simulink model "chris_1R_hsv_vortex_follow"  (R2024b)
settings: Solver=FixedStepDiscrete  StartTime=0.0  StopTime=20  FixedStep=0.1  MaxStep=0.1  RelTol=1e-3
libraries: realtime_pacer_lib x1
settings Model: Creator=RSL  LastModifiedBy=cwaight
settings SolverCC: AlgebraicLoopSolver=TrustRegion
settings DataIOCC: ReturnWorkspaceOutputs=off
settings DebuggingCC: UnconnectedInputMsg=warning  UnconnectedOutputMsg=warning  UnconnectedLineMsg=warning  ArithmeticOperatorsInVariantConditions=warning
settings ModelReferenceCC: EnableRefExpFcnMdlSchedulingChecks=on
settings SFSimCC: SimUseLocalCustomCode=off  CustomCodeUndefinedFunction=UseInterfaceOnly
settings RTWCC: RTWUseLocalCustomCode=off  GPUComputeCapability=3.5
settings CodeAppCC: StateflowObjectComments=on

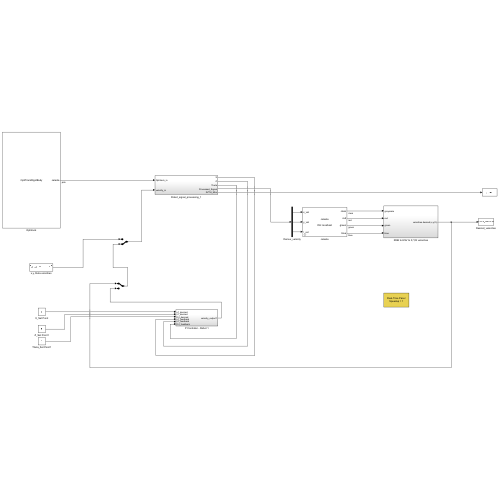
[thumbnail: Simulink's stored preview of the top-level diagram]
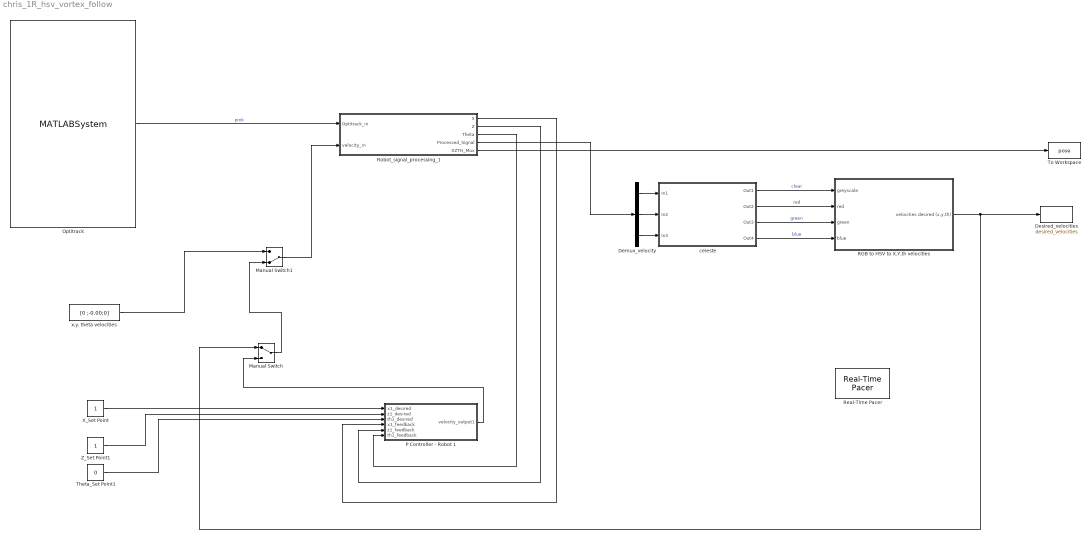
== system chris_1R_hsv_vortex_follow ==
  Demux_velocity : Demux  Outputs=3
  Desired_velocities : ToWorkspace  VariableName=desired_velocities  SampleTime=-1
  Manual Switch : ManualSwitch
  Manual Switch1 : ManualSwitch  CurrentSetting=0
  Optitrack : MATLABSystem  System=OptiTrackRigidBody  coordinateTransformationMatrix=[ 1, 0, 0; 0, 0, 1; 0, -1, 0 ]  rigidBodyNames={ 'celeste'}  orientationFormat=Euler angles  debug=on  natNetHostAddress=127.0.0.1  natNetClientAddress=127.0.0.1  dllPath=C:\DecaMATLAB\NatNetSDK\lib\x64\NatNetML.dll  unicast=off
      mask Type: OptiTrackRigidBody
      mask Display:
      | disp('OptiTrackRigidBody');
      | port_label('output',1,'celeste');
  P Controller - Robot 1 : Subsystem
  RGB to HSV to X,Y,th velocities : Subsystem
  Real-Time Pacer : realtime_pacer_lib/Real-Time Pacer  simTimePerRealTime=1
  Robot_signal_processing_1 : Subsystem
  "Theta_Set Point1 " : Constant  Value=0
  To Workspace : ToWorkspace  VariableName=pose  SampleTime=-1
  X_Set Point : Constant
  Z_Set Point1 : Constant
  celeste : Subsystem  mask(DecabotMask){robotName=celeste, decabotHelper=localhost, robotAddress=, useDataTurbine=off, useDirectSocket=on, debug=off}
      mask prompts: robotName "Robot name:"; decabotHelper "DecabotHelper/DataTurbine server:"; robotAddress "Robot network address (optional):"; useDataTurbine "Use DataTurbine"; useDirectSocket "Use direct robot TCP connection"; debug "Log debug messages"
      mask help: This is a masked subsystem that contains a Decabot block for bidirectional communication with a decabot over a direct TCP socket connection.
      mask init:
      | robotName = 'Nobody';
      | decabotHelper = 'localhost';
      | robotAddress = '';
      | useDataTurbine = true;
      | debug = true;
      mask TypeOptions robotName: decabot/robotName
      mask Callback robotName:
      | try
      |     set_param( gcb( ), 'Name', get_param( gcb( ), 'robotName' ) );
      | end
      mask TypeOptions decabotHelper: decabot/decabotHelper
      mask TypeOptions robotAddress: decabot/robotAddress
      mask TypeOptions useDataTurbine: decabot/useDataTurbine
      mask TypeOptions useDirectSocket: decabot/useDirectSocket
      mask TypeOptions debug: decabot/debug
      mask Display:
      | disp( [get_param( gcb( ), 'robotName' ) '\n\nDH: ' get_param( gcb( ), 'decabotHelper' ) ] );
      | 
      | port_label('input',1,'x_vel');
      | port_label('input',2,'y_vel');
      | port_label('input',3,'t_vel');
      | 
      | port_label('output',1,'clear');
      | port_label('output',2,'red');
      | port_label('output',3,'green');
      | port_label('output',4,'blue');
  "x,y, theta velocities" : Constant  Value=[0 ;-0.00;0]
  wires:
  Demux_velocity/3 -> celeste/3(In3)
  Demux_velocity/1 -> celeste/1(In1)
  Demux_velocity/2 -> celeste/2(In2)
  X_Set Point/1 -> P Controller - Robot 1/1(x1_desired)
  Z_Set Point1/1 -> P Controller - Robot 1/2(z1_desired)
  "Theta_Set Point1 "/1 -> P Controller - Robot 1/3(th1_desired)
  Robot_signal_processing_1/3(Theta) -> P Controller - Robot 1/6(th1_feedback)
  Robot_signal_processing_1/2(Z) -> P Controller - Robot 1/5(z1_feedback)
  Robot_signal_processing_1/1(X) -> P Controller - Robot 1/4(x1_feedback)
  Optitrack/1 -> Robot_signal_processing_1/1(Optitrack_in)  "pink"
  Robot_signal_processing_1/4(Processed_Signal) -> Demux_velocity/1
  celeste/1(Out1) -> RGB to HSV to X,Y,th velocities/1(greyscale)  "clear"
  celeste/2(Out2) -> RGB to HSV to X,Y,th velocities/2(red)  "red"
  celeste/3(Out3) -> RGB to HSV to X,Y,th velocities/3(green)  "green"
  celeste/4(Out4) -> RGB to HSV to X,Y,th velocities/4(blue)  "blue"
  Manual Switch1/1 -> Robot_signal_processing_1/2(velocity_in)
  P Controller - Robot 1/1(velocity_output1) -> Manual Switch/2
  Manual Switch/1 -> Manual Switch1/2
  "x,y, theta velocities"/1 -> Manual Switch1/1
  RGB to HSV to X,Y,th velocities/1(velocities desired (x,y,th)) -> Desired_velocities/1, Manual Switch/1
  Robot_signal_processing_1/5(XZTH_Mux) -> To Workspace/1

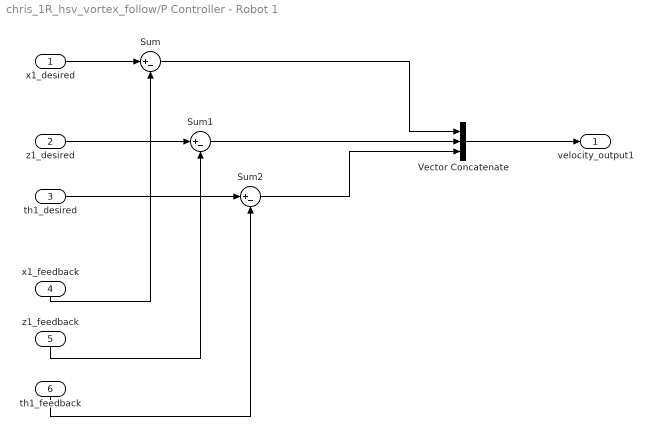
== system chris_1R_hsv_vortex_follow/P Controller - Robot 1 ==
  x1_desired : Inport
  z1_desired : Inport  Port=2
  th1_desired : Inport  Port=3
  x1_feedback : Inport  Port=4
  z1_feedback : Inport  Port=5
  th1_feedback : Inport  Port=6
  Sum : Sum  Inputs=|+-
  Sum1 : Sum  Inputs=|+-
  Sum2 : Sum  Inputs=|+-
  Vector Concatenate : Concatenate  NumInputs=3
  velocity_output1 : Outport
  wires:
  Vector Concatenate/1 -> velocity_output1/1
  x1_desired/1 -> Sum/1
  Sum/1 -> Vector Concatenate/1
  th1_feedback/1 -> Sum2/2
  x1_feedback/1 -> Sum/2
  z1_feedback/1 -> Sum1/2
  Sum2/1 -> Vector Concatenate/3
  th1_desired/1 -> Sum2/1
  Sum1/1 -> Vector Concatenate/2
  z1_desired/1 -> Sum1/1

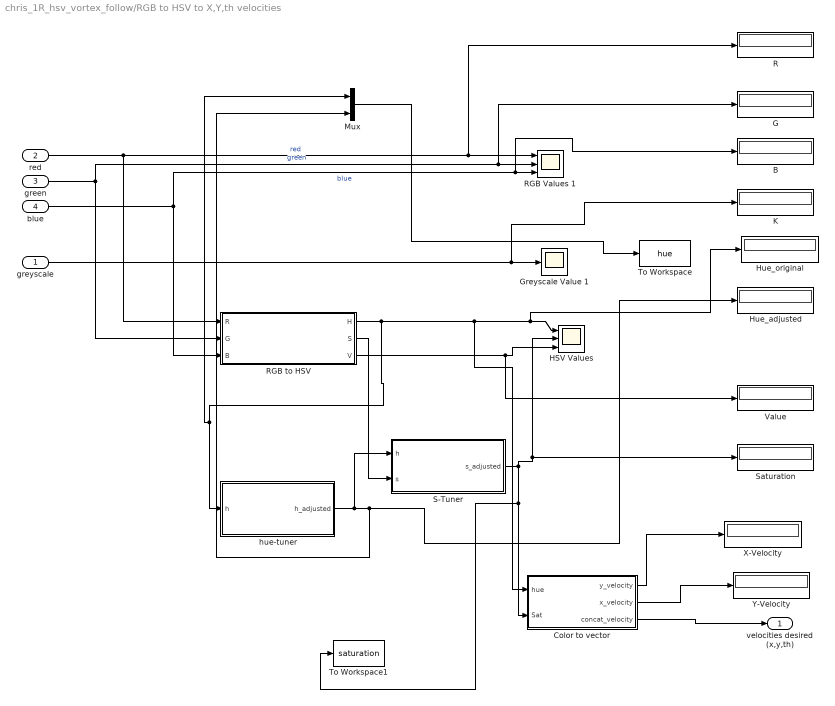
== system chris_1R_hsv_vortex_follow/RGB to HSV to X,Y,th velocities ==
  greyscale : Inport
  red : Inport  Port=2
  green : Inport  Port=3
  blue : Inport  Port=4
  B : Display
  Color to vector : Subsystem
  G : Display
  Greyscale Value 1 : Scope
  HSV Values : Scope  NumInputPorts=3
  Hue_adjusted : Display
  Hue_original : Display
  K : Display
  Mux : Mux  Inputs=2
  R : Display
  "RGB Values 1 " : Scope  NumInputPorts=3
  RGB to HSV : MATLAB Function  TreatAsAtomicUnit=on
  S-Tuner : MATLAB Function  TreatAsAtomicUnit=on
  Saturation : Display
  To Workspace : ToWorkspace  VariableName=hue  SaveFormat=Timeseries  SampleTime=-1
  To Workspace1 : ToWorkspace  VariableName=saturation  SaveFormat=Timeseries  SampleTime=-1
  Value : Display
  X-Velocity : Display
  "Y-Velocity " : Display
  hue-tuner : MATLAB Function  TreatAsAtomicUnit=on
  velocities desired (x,y,th) : Outport
  wires:
  red/1 -> R/1, "RGB Values 1 "/1, RGB to HSV/1(R)  "red"
  blue/1 -> B/1, "RGB Values 1 "/3, RGB to HSV/3(B)  "blue"
  greyscale/1 -> K/1, Greyscale Value 1/1
  green/1 -> G/1, "RGB Values 1 "/2, RGB to HSV/2(G)  "green"
  RGB to HSV/3(V) -> Value/1, HSV Values/3
  RGB to HSV/2(S) -> S-Tuner/2(s)
  S-Tuner/1(s_adjusted) -> HSV Values/2, Saturation/1, To Workspace1/1, Color to vector/2(Sat)
  Color to vector/1(y_velocity) -> X-Velocity/1
  Color to vector/2(x_velocity) -> "Y-Velocity "/1
  Color to vector/3(concat_velocity) -> velocities desired (x,y,th)/1
  hue-tuner/1(h_adjusted) -> S-Tuner/1(h), Mux/2, Hue_adjusted/1
  Mux/1 -> To Workspace/1
  RGB to HSV/1(H) -> Color to vector/1(hue), Hue_original/1, HSV Values/1, Mux/1, hue-tuner/1(h)

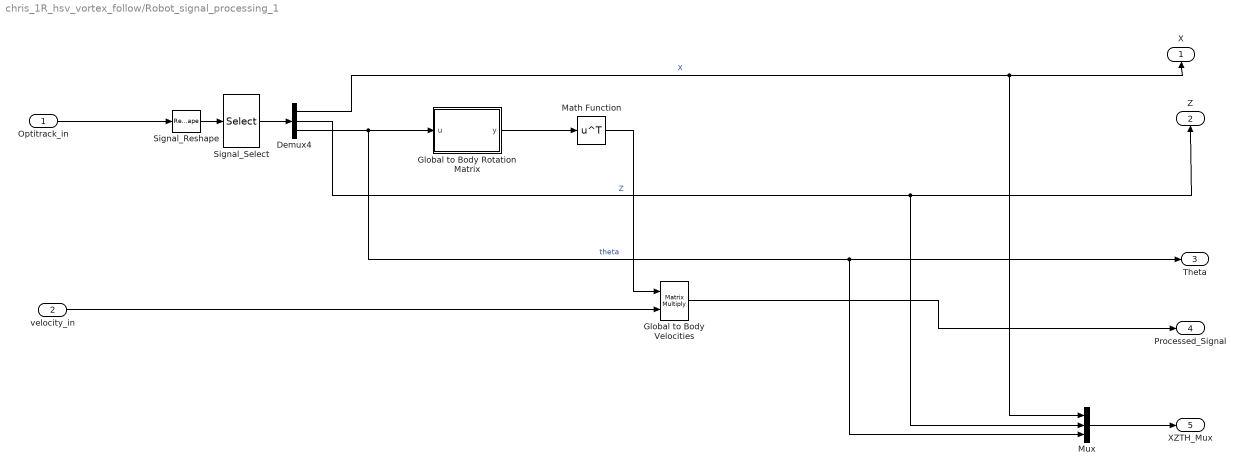
== system chris_1R_hsv_vortex_follow/Robot_signal_processing_1 ==
  Optitrack_in : Inport
  velocity_in : Inport  Port=2
  Demux4 : Demux  Outputs=3
  Global to Body Velocities : Product  Multiplication=Matrix(*)
  Global to Body Rotation Matrix : MATLAB Function  TreatAsAtomicUnit=on
  Math Function : Math  Operator=transpose  SignedPower=on
  Mux : Mux  Inputs=3
  Signal_Reshape : Reshape  OutputDimensions=6
  Signal_Select : Selector  InputPortWidth=6  IndexOptions=Index vector (dialog)  Indices=[1 2 6]  OutputSizes=1
  X : Outport
  Z : Outport  Port=2
  Theta : Outport  Port=3
  Processed_Signal : Outport  Port=4
  XZTH_Mux : Outport  Port=5
  wires:
  Demux4/1 -> Mux/1, X/1  "X"
  Demux4/3 -> Mux/3, Theta/1, Global to Body Rotation Matrix/1(u)  "theta"
  Demux4/2 -> Mux/2, Z/1  "Z"
  Global to Body Velocities/1 -> Processed_Signal/1
  Signal_Reshape/1 -> Signal_Select/1
  velocity_in/1 -> Global to Body Velocities/2
  Optitrack_in/1 -> Signal_Reshape/1
  Global to Body Rotation Matrix/1(y) -> Math Function/1
  Signal_Select/1 -> Demux4/1
  Math Function/1 -> Global to Body Velocities/1
  Mux/1 -> XZTH_Mux/1

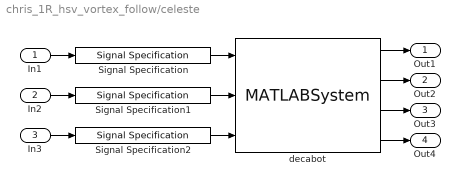
== system chris_1R_hsv_vortex_follow/celeste ==
  In1 : Inport
  In2 : Inport  Port=2
  In3 : Inport  Port=3
  Signal Specification : SignalSpecification  OutDataTypeStr=double  Dimensions=1
  Signal Specification1 : SignalSpecification  OutDataTypeStr=double  Dimensions=1
  Signal Specification2 : SignalSpecification  OutDataTypeStr=double  Dimensions=1
  decabot : MATLABSystem  System=Decabot  robotName=celeste  decabotHelper=localhost  useDataTurbine=off  useDirectSocket=on  debug=off
      mask Type: Decabot
      mask Display:
      | disp('celeste\n\nDH: localhost');
      | port_label('input',1,'x_vel');
      | port_label('input',2,'y_vel');
      | port_label('input',3,'t_vel');
      | port_label('output',1,'clear');
      | port_label('output',2,'red');
      | port_label('output',3,'green');
      | port_label('output',4,'blue');
  Out1 : Outport
  Out2 : Outport  Port=2
  Out3 : Outport  Port=3
  Out4 : Outport  Port=4
  wires:
  Signal Specification2/1 -> decabot/3
  Signal Specification1/1 -> decabot/2
  Signal Specification/1 -> decabot/1
  In2/1 -> Signal Specification1/1
  decabot/4 -> Out4/1
  decabot/1 -> Out1/1
  decabot/3 -> Out3/1
  decabot/2 -> Out2/1
  In1/1 -> Signal Specification/1
  In3/1 -> Signal Specification2/1

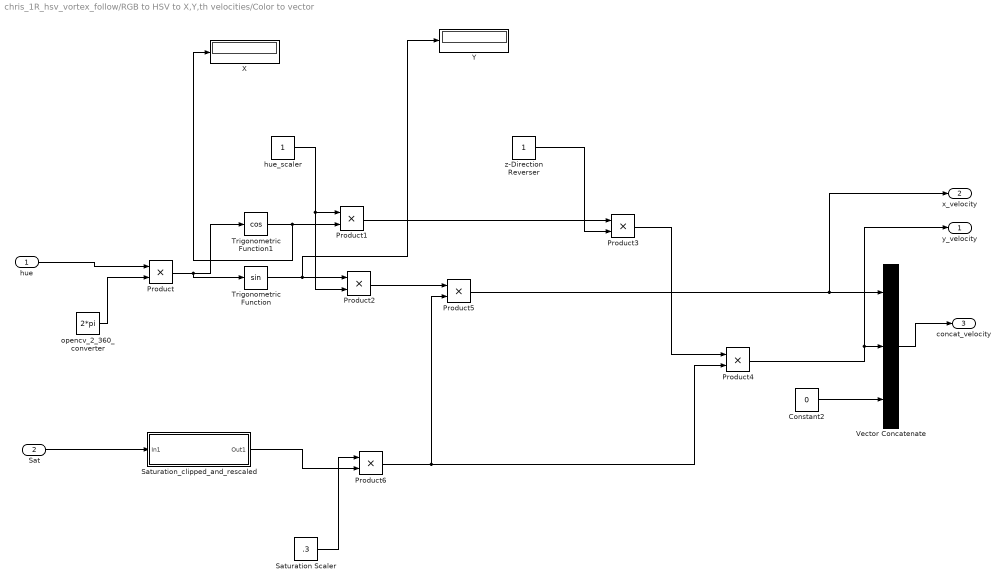
== system chris_1R_hsv_vortex_follow/RGB to HSV to X,Y,th velocities/Color to vector ==
  hue : Inport
  Sat : Inport  Port=2
  Constant2 : Constant  Value=0
  Product{,1..6} (7 alike) : Product
  Saturation Scaler : Constant  Value=.3
  Saturation_clipped_and_rescaled : Subsystem
  Trigonometric Function : Trigonometry
  Trigonometric Function1 : Trigonometry  Operator=cos
  Vector Concatenate : Concatenate  NumInputs=3
  X : Display
  Y : Display
  hue_scaler : Constant
  opencv_2_360_converter : Constant  Value=2*pi
  z-Direction Reverser : Constant
  y_velocity : Outport
  x_velocity : Outport  Port=2
  concat_velocity : Outport  Port=3
  wires:
  Trigonometric Function/1 -> Y/1, Product2/1
  opencv_2_360_converter/1 -> Product/2
  Product2/1 -> Product5/1
  Trigonometric Function1/1 -> X/1, Product1/2
  Product/1 -> Trigonometric Function1/1, Trigonometric Function/1
  Product1/1 -> Product3/1
  hue/1 -> Product/1
  hue_scaler/1 -> Product2/2, Product1/1
  Vector Concatenate/1 -> concat_velocity/1
  z-Direction Reverser/1 -> Product3/2
  Product3/1 -> Product4/1
  Product5/1 -> x_velocity/1, Vector Concatenate/1
  Constant2/1 -> Vector Concatenate/3
  Saturation Scaler/1 -> Product6/1
  Product6/1 -> Product4/2, Product5/2
  Product4/1 -> y_velocity/1, Vector Concatenate/2
  Sat/1 -> Saturation_clipped_and_rescaled/1(In1)
  Saturation_clipped_and_rescaled/1(Out1) -> Product6/2

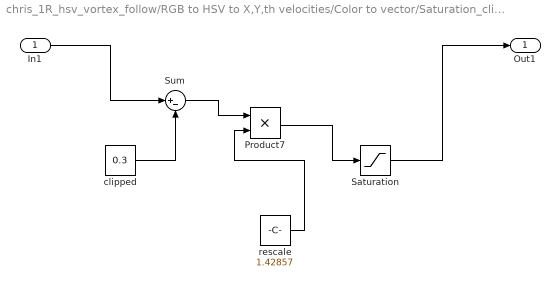
== system chris_1R_hsv_vortex_follow/RGB to HSV to X,Y,th velocities/Color to vector/Saturation_clipped_and_rescaled ==
  In1 : Inport
  Product7 : Product
  Saturation : Saturate  UpperLimit=1  LowerLimit=0.05
  Sum : Sum  Inputs=|+-
  clipped : Constant  Value=0.3
  rescale : Constant  Value=1.42857
  Out1 : Outport
  wires:
  clipped/1 -> Sum/2
  Saturation/1 -> Out1/1
  In1/1 -> Sum/1
  Product7/1 -> Saturation/1
  rescale/1 -> Product7/2
  Sum/1 -> Product7/1

== matlab function chris_1R_hsv_vortex_follow/RGB to HSV to X,Y,th velocities/RGB to HSV ==
  data: R input; H output; G input; B input; S output; V output
function [H, S, V]= rgb2hsv_func(R, G, B)

% This one is tuned for the robot - pink

  % Clip RGB values to be within the range [100, 1200]
  R = max(min(R, 1800), 200);
  G = max(min(G, 2200), 250);
  B = max(min(B, 1900), 250);

  % Normalize RGB to [0, 1]
  R = (R - 200) / (1800-200); 
  G = (G - 250) / (2200-250);
  B = (B - 250) / (1900-250);

  Cmax = max(max(R, G), B);
  Cmin = min(min(R, G), B);
  delta = Cmax - Cmin;

  H = zeros(size(R));
  S = zeros(size(R));
  V = Cmax;

  % Calculate Hue
  ind = find(delta ~= 0); 
  r_ind = find((Cmax == R) & (delta ~= 0));
  g_ind = find((Cmax == G) & (delta ~= 0));
  b_ind = find((Cmax == B) & (delta ~= 0));

  H(r_ind) = 60 * mod((G(r_ind) - B(r_ind)) ./ delta(r_ind), 6);
  H(g_ind) = 60 * (((B(g_ind) - R(g_ind)) ./ delta(g_ind)) + 2);
  H(b_ind) = 60 * (((R(b_ind) - G(b_ind)) ./ delta(b_ind)) + 4);

  H = H / 360;

  % Calculate Saturation
  S(ind) = delta(ind) ./ Cmax(ind);

end

== matlab function chris_1R_hsv_vortex_follow/RGB to HSV to X,Y,th velocities/S-Tuner ==
  data: h input; s_adjusted output; s input
function s_adjusted   = saturation_adjust(h,s)
    if 0 <= h && h <= 0.05
        s_adjusted = max(0, (s - 0.1114) * (0.7/0.9129) ) + 0.3;
    elseif 0.05 <= h && h <= 0.1
        s_adjusted = max(0, (s - 0.1915) * (0.7/0.665)) + 0.3;
    elseif 0.1 <= h && h <= 0.15
        s_adjusted = max(0, (s - 0.1613) * (0.7/0.6136)) + 0.3;
    elseif 0.15 <= h && h <= 0.2
        s_adjusted = max(0, (s - 0.1096) * (0.7/0.6058)) + 0.3;
    elseif 0.2 <= h && h <= 0.25
        s_adjusted = max(0, (s - 0.0677) * (0.7/0.5851)) + 0.3;
        
    elseif 0.25 <= h && h <= 0.3
        s_adjusted = max(0, (s + 0.1056) * (0.7/0.7955)) + 0.3;
    elseif 0.3 <= h && h <= 0.35
        s_adjusted = max(0, (s + 0.0671) * (0.7/0.644)) + 0.3;
    elseif 0.35 <= h && h <= 0.4
        s_adjusted = max(0, (s - 0.0036) * (0.7/0.3670)) + 0.3;
    elseif 0.4 <= h && h <= 0.45
        s_adjusted = max(0, (s - 0.0768) * (0.7/0.2182)) + 0.3;
    elseif 0.45 <= h && h <= 0.5
        s_adjusted = max(0, (s - 0.0453) * (0.7/0.4158)) + 0.3;

    elseif 0.5 <= h && h <= 0.55
        s_adjusted = max(0, (s - 0.0776) * (0.7/0.4708)) + 0.3;
    elseif 0.55 <= h && h <= 0.6
        s_adjusted = max(0, (s + 0.19) * (0.7/1.1235)) + 0.3;
    elseif 0.6 <= h && h <= 0.65
        s_adjusted = max(0, (s + 0.0663) * (0.7/0.9176)) + 0.3;
    elseif 0.65 <= h && h <= 0.7
        s_adjusted = max(0, (s - 0.0246) * (0.7/0.6231)) + 0.3;
    elseif 0.7 <= h && h <= 0.75
        s_adjusted = max(0, (s - 0.0774) * (0.7/0.5134)) + 0.3;       
        
    elseif 0.75 <= h && h <= 0.8
        s_adjusted = max(0, (s - 0.1307) * (0.7/0.4236)) + 0.3;
    elseif 0.8 <= h && h <= 0.85
        s_adjusted = max(0, (s - 0.2109) * (0.7/0.4814)) + 0.3;
    elseif 0.85 <= h && h <= 0.9
        s_adjusted = max(0, (s - 0.1347) * (0.7/0.7503)) + 0.3;
    elseif 0.9 <= h && h <= 0.95
        s_adjusted = max(0, (s - 0.0922) * (0.7/0.9583)) + 0.3;
    elseif 0.95 <= h && h <= 1
        s_adjusted = max(0, (s - 0.0796) * (0.7/1.0081)) + 0.3;
                
    else
        s_adjusted = s;  
    end
    
    s_adjusted = min(1, s_adjusted);
end

== matlab function chris_1R_hsv_vortex_follow/Robot_signal_processing_1/Global to Body Rotation Matrix ==
  data: u input; y output
function y = fcn(u)

y = [cos(u) -sin(u) 0; sin(u) cos(u) 0; 0 0 1];

== matlab function chris_1R_hsv_vortex_follow/RGB to HSV to X,Y,th velocities/hue-tuner ==
  data: h input; h_adjusted output
function h_adjusted   = hue_adjust(h)
    if 0.021 <= h && h <= 0.3
        h_adjusted = max(0, (h + 0.0207) * 1/0.739);
    elseif 0.3 <= h && h <= 0.5
        h_adjusted = max(0, (h + 0.5696) * 1/2.4058);
    elseif 0.5 <= h && h <= 0.7
        h_adjusted = max(0, h - 0.3632) * 1/0.4533 ;
    elseif 0.7 <= h && h <= .85
        h_adjusted = max(0, (h + 0.498) * 1/1.7413) ;
    elseif 0.85 <= h && h <= 1
        h_adjusted = max(0, (h - 0.6648) * 1/0.3342);
    else
        h_adjusted = h;
    end
    
    h_adjusted = min(1, h_adjusted);
end
